simulink model "Switch"  (R2015b)
settings: Solver=VariableStepAuto  StartTime=0.0  StopTime=10.0  RelTol=1e-3
settings Model: Creator=LUBO  LastModifiedBy=LUBO

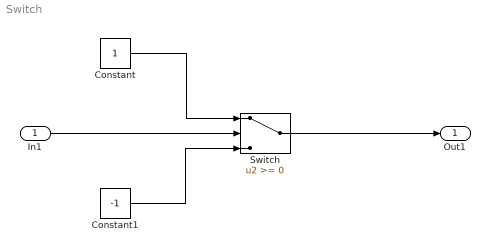
== system Switch ==
  In1 : Inport
  Constant : Constant
  Constant1 : Constant  Value=-1
  Switch : Switch
  Out1 : Outport
  wires:
  Constant/1 -> Switch/1
  Constant1/1 -> Switch/3
  In1/1 -> Switch/2
  Switch/1 -> Out1/1
